simulink model "state_test"  (R2015a)
settings: Solver=ode4  StartTime=0.0  StopTime=5  FixedStep=0.01  RelTol=1e-3
values from neighbouring files (symbols this model uses):
  A = [0 1 0 0 ... (first row only)    [following.m]    (also in hoge.m = [0 1; servo.m)
  B = [0 2 0 0]'    [following.m]    (also in hoge.m = [0 1]'; servo.m)
  C = eye(4)    [following.m]    (also in hoge.m = [1 0]; servo.m)
  D = zeros(4,1)    [following.m]    (also in hoge.m = 0; servo.m)
  x0 = zeros(4,1)    [following.m]    (also in hoge.m = [1 0]'; servo.m)
settings Model: Creator=shohei  LastModifiedBy=shohei

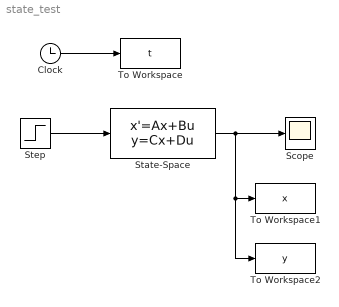
== system state_test ==
  Clock : Clock
  Scope : Scope
  State-Space : StateSpace  A=A  B=B  C=C  D=D  X0=x0
  Step : Step  Time=0  SampleTime=0
  To Workspace : ToWorkspace  VariableName=t  SampleTime=-1
  To Workspace1 : ToWorkspace  VariableName=x  SampleTime=-1
  To Workspace2 : ToWorkspace  VariableName=y  SampleTime=-1
  wires:
  Clock/1 -> To Workspace/1
  State-Space/1 -> To Workspace2/1, To Workspace1/1, Scope/1
  Step/1 -> State-Space/1
